simulink model "nldemo_master"  (R2020b)
settings: Solver=FixedStepAuto  StartTime=0.0  StopTime=inf  FixedStep=0.01  RelTol=1e-3
undefined symbols (not defined in the file): autopilot, control, kspTxIn0, P_m_rocket, P_x_target
libraries: ksplib x3
settings Model: DataDictionary=kspdemo.sldd  EnablePacing=on  PacingRate=2  Creator=brianhannan  LastModifiedBy=wizard

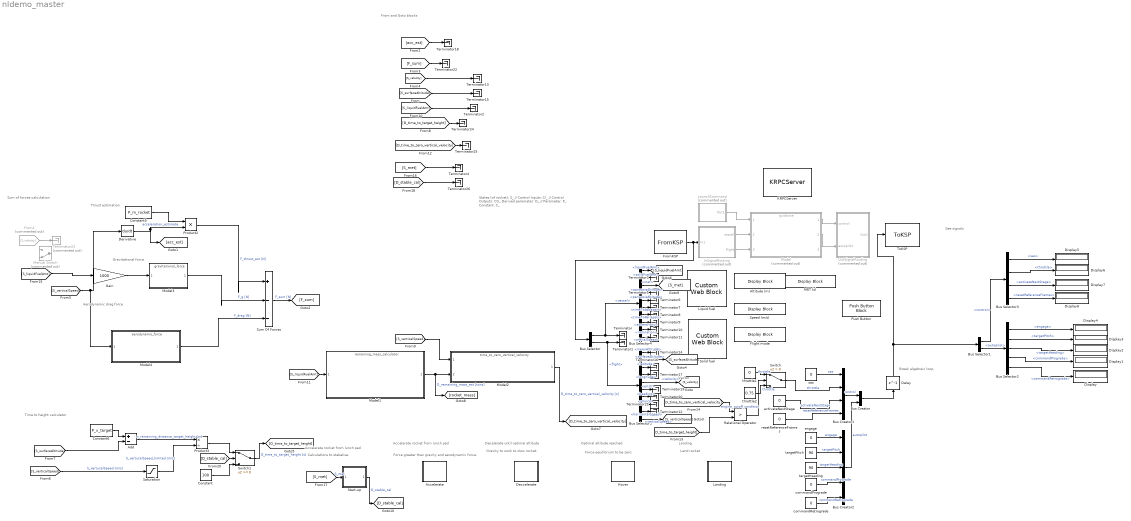
== system nldemo_master ==
  note: Time to height calculator
  note: Vector
  note: From and Goto blocks
  note: Thrust estimation
  note: States (of rocket): 		S_         //
      | Control Inputs: 		CI_       //
      | Control Outputs:		CO_
      | Derived parameter: 	D_     //
      | Parameter:				P_
      | Constant:				C_
  note: Gravitational force
  note: Sum of forces calculation
  note: Gravity to work to slow rocket.
  note: Decelerate until optimal altitude
  note: See signals
  note: Break algebraic loop
  note: Optimal altitude reached
  note: Accelerate rocket from lunch pad
  note: Force greater than gravity and aerodynamic force.
  note: Force equilibrium to be zero:
  note: Land rocket
  note: Landing
  note: Aerodynamic drag force
  note: Accelerate rocket from lunch pad
  note: Calculations to stabalise.
  Accelerate : Stateflow chart  TreatAsAtomicUnit=on
  Add : Sum  Inputs=+-
  Altitude (m) : DisplayBlock  LabelPosition=Bottom  Format=short  Transparency=1
  Bus Creator : BusCreator  Inputs=2  OutDataTypeStr=Bus: kspTxIn  NonVirtualBus=on
  Bus Creator1 : BusCreator  Inputs=4  OutDataTypeStr=Bus: control  NonVirtualBus=on
  Bus Creator2 : BusCreator  Inputs=5  OutDataTypeStr=Bus: autopilot  NonVirtualBus=on
  Bus Selector : BusSelector  OutputSignals=vessel,flight
  Bus Selector1 : BusSelector  OutputSignals=control,autopilot
  Bus Selector2 : BusSelector  OutputSignals=engage,targetPitch,targetHeading,commandPrograde,commandRetrograde
  Bus Selector3 : BusSelector  OutputSignals=sas,throttle,activateNextStage,resetReferenceFrames
  Bus Selector4 : BusSelector  OutputSignals=liquidFuelAmt,solidFuelAmt,met,apoapsisAltitude,periapsisAltitude,timeToApoapsis,timeToPeriapsis,eccentricity,inclination,orbitalSpeed
  Bus Selector5 : BusSelector  OutputSignals=meanAltitude,surfaceAltitude,latitude,longitude,velocity,pitch,heading,gForce,horizontalSpeed,verticalSpeed
  Constant : Constant  Value=100
  Constant5 : Constant  Value=P_m_rocket
  Constant6 : Constant  Value=P_x_target
  "Deccelerate " : Stateflow chart  TreatAsAtomicUnit=on
  Delay : Delay  DelayLength=1
  Derivative : Derivative
  Display{,1..8} (9 alike) : Display
  Flight mode : DisplayBlock  LabelPosition=Bottom  Format=short  Transparency=1
  From1 : From  Commented=on  GotoTag=S_velocity
  FromKSP : ksplib/FromKSP
  Gain : Gain  Gain=1000
  Hover : Stateflow chart  TreatAsAtomicUnit=on
  InSignalRouting : Subsystem  Commented=on
  KRPCServer : ksplib/KRPCServer
  Landing : Stateflow chart  TreatAsAtomicUnit=on
  LaunchCommand : Subsystem  Commented=on  mask(Launch Command){launchCmd=logical(0)}
      mask prompts: launchCmd "Launch:"
      mask help: Send launch command
      mask Display: disp('Launch')
  Liquid fuel : CustomWebBlock  LabelPosition=Hide  ShowInitialText=on  Configuration="{\"components\":[{\"name\":\"CircularScaleComponent\",\"settings\":{\"bounds\":{\"max\":225,\"min\":0,\"tickInterval\":\"auto\"},\"direction\":\"cw\",\"flipLimits\":0,\"innerRadius\":0.75,\"internalTickHeightScaleFactor\":1,\"labelColor\":[255,252,199],\"labelFont\":{\"font\":\"Arial\",\"fontSize\":12},\"labelTransparency\":1,\"minorTickHeightScaleFactor\":0.2,\"needleImage\":{\"size\":[1890,567],\"src\":\"data:image\\/svg+xml;base64,PD94bWwgdmVyc2lvbj0iMS4wIiBlbmNvZGluZz0iVVRGLTgiIHN0YW5kYWxvbmU9Im5vIj8+CjxzdmcKICAgeG1sbnM6ZGM9Imh0dHA6Ly9wdXJsLm9yZy9kYy9lbGVtZW50cy8xLjEvIgogICB4bWxuczpjYz0iaHR0cDovL2NyZWF0aXZlY29tbW9ucy5vcmcvbnMjIgogICB4bWxuczpyZGY9Imh0dHA6Ly93d3cudzMub3JnLzE5OTkvMDIvMjItcmRmLXN5bnRheC1ucyMiCiAgIHhtbG5zOnN2Zz0iaHR0cDovL3d3dy53My5vcmcvMjAwMC9zdmciCiAgIHhtbG5zPSJodHRwOi8vd3d3LnczLm9yZy8yMDAwL3N2ZyIKICAgeG1sbnM6 ...(+4096 chars)\"},\"needleOffset\":[0.1610917094974375,0],\"needleOrientation\":-45,\"needleRotation\":180.59702388394928,\"needleSize\":{\"height\":0.13032601008944536,\"width\":0.416859542883425},\"outerRadius\":0.9,\"position\":[0.06486742424242424,0.05627705627705628,0.8917748917748918,0.8787878787878788],\"scaleAngle\":270,\"scaleAngleOffset\":135,\"scaleColors\":[],\"scaleColorsSize\":0.2,\"scalePosition\":[0,0,1,1],\"showLabels\":1,\"showMinorTicks\":1,\"showSpanLine\":1,\"showTicks\":1,\"tickColor\":[255,255,200],\"tickTransparency\":1,\"valueBarColor\":[0,114,189],\"valueBarPosition\":[0,0,1,1],\"valueBarSize\":0.2,\"valueBarTransparency\":1}},{\"name\":\"BackgroundImageComponent\",\"settings\":{\"image\":{\"size\":[500,500],\"src\":\"data:image\\/svg+xml;base64,PD94bWwgdmVyc2lvbj0iMS4wIiBlbmNvZGluZz0iVVRGLTgiIHN0YW5kYWxvbmU9Im5vIj8+CjxzdmcKICAgeG1sbnM6ZGM9Imh0dHA6Ly9wdXJsLm9yZy9kYy9lbGVtZW50cy8xLjEvIgogICB4bWxuczpjYz0iaHR0cDovL2NyZWF0aXZlY29tbW9ucy5vcmcvbnMjIgogICB4bWxuczpyZGY9Imh0dHA6Ly93d3cudzMub3JnLzE5OTkvMDIvMjItcmRmLXN5bnRheC1ucyMiCiAgIHhtbG5zOnN2Zz0iaHR0cDovL3d3dy53My5vcmcvMjAwMC9zdmciCiAgIHhtbG5zPSJodHRwOi8vd3d3LnczLm9yZy8yMDAwL3N2ZyIKICAgeG1sbnM6 ...(+9964 chars)\"},\"position\":[0,0,1,1],\"scaleMode\":\"0\"}},{\"name\":\"ForegroundImageComponent\",\"settings\":{\"image\":{\"size\":[0,0],\"src\":\"default\",\"srcOrientation\":[]},\"isForeground\":1,\"position\":[0,0,1,1],\"scaleMode\":\"0\"}}],\"settings\":{\"BindingType\":\"signal\",\"aspectRatio\":1.0318471337579618,\"direction\":\"cw\",\"fixedAspectRatio\":\"on\",\"flipLimits\":0,\"orientation\":\"horizontal\"},\"type\":\"CircularGauge\"}"
  MET (s) : DisplayBlock  LabelPosition=Bottom  Format=short  Transparency=1
  Manual Switch : ManualSwitch  Commented=on  CurrentSetting=0
  Model : ModelReference  Commented=on  ModelNameDialog=guidance  SimulationMode=Normal  ModelReferenceVersion=1.177
  Model1 : ModelReference  ModelNameDialog=remaining_mass_calculator.slx  SimulationMode=Normal  ModelReferenceVersion=1.2
  Model2 : ModelReference  ModelNameDialog=time_to_zero_vertical_velocity.slx  SimulationMode=Normal  ModelReferenceVersion=1.4
  Model3 : ModelReference  ModelNameDialog=gravitational_force.slx  SimulationMode=Normal  ModelReferenceVersion=1.5
  Model4 : ModelReference  ModelNameDialog=aerodynamic_force.slx  SimulationMode=Normal  ModelReferenceVersion=1.5
  OutSignalRouting : Subsystem  Commented=on
  Product2 : Product
  Product3 : Product  Inputs=*/
  Push Button : PushButtonBlock  ButtonText=Launch
  Relational Operator : RelationalOperator  Operator=>  OutDataTypeStr=boolean  RndMeth=Simplest
  Saturation : Saturate  UpperLimit=10000  LowerLimit=0.0001
  Solid fuel : CustomWebBlock  LabelPosition=Hide  ShowInitialText=on  Configuration="{\"components\":[{\"name\":\"CircularScaleComponent\",\"settings\":{\"bounds\":{\"max\":750,\"min\":0,\"tickInterval\":\"auto\"},\"direction\":\"cw\",\"flipLimits\":0,\"innerRadius\":0.75,\"internalTickHeightScaleFactor\":1,\"labelColor\":[255,252,199],\"labelFont\":{\"font\":\"Arial\",\"fontSize\":12},\"labelTransparency\":1,\"minorTickHeightScaleFactor\":0.2,\"needleImage\":{\"size\":[1890,567],\"src\":\"data:image\\/svg+xml;base64,PD94bWwgdmVyc2lvbj0iMS4wIiBlbmNvZGluZz0iVVRGLTgiIHN0YW5kYWxvbmU9Im5vIj8+CjxzdmcKICAgeG1sbnM6ZGM9Imh0dHA6Ly9wdXJsLm9yZy9kYy9lbGVtZW50cy8xLjEvIgogICB4bWxuczpjYz0iaHR0cDovL2NyZWF0aXZlY29tbW9ucy5vcmcvbnMjIgogICB4bWxuczpyZGY9Imh0dHA6Ly93d3cudzMub3JnLzE5OTkvMDIvMjItcmRmLXN5bnRheC1ucyMiCiAgIHhtbG5zOnN2Zz0iaHR0cDovL3d3dy53My5vcmcvMjAwMC9zdmciCiAgIHhtbG5zPSJodHRwOi8vd3d3LnczLm9yZy8yMDAwL3N2ZyIKICAgeG1sbnM6 ...(+4096 chars)\"},\"needleOffset\":[0.1610917094974375,0],\"needleOrientation\":-45,\"needleRotation\":180.59702388394928,\"needleSize\":{\"height\":0.13032601008944536,\"width\":0.416859542883425},\"outerRadius\":0.9,\"position\":[0.06486742424242424,0.05627705627705628,0.8917748917748918,0.8787878787878788],\"scaleAngle\":270,\"scaleAngleOffset\":135,\"scaleColors\":[],\"scaleColorsSize\":0.2,\"scalePosition\":[0,0,1,1],\"showLabels\":1,\"showMinorTicks\":1,\"showSpanLine\":1,\"showTicks\":1,\"tickColor\":[255,255,200],\"tickTransparency\":1,\"valueBarColor\":[0,114,189],\"valueBarPosition\":[0,0,1,1],\"valueBarSize\":0.2,\"valueBarTransparency\":1}},{\"name\":\"BackgroundImageComponent\",\"settings\":{\"image\":{\"size\":[500,500],\"src\":\"data:image\\/svg+xml;base64,PD94bWwgdmVyc2lvbj0iMS4wIiBlbmNvZGluZz0iVVRGLTgiIHN0YW5kYWxvbmU9Im5vIj8+CjxzdmcKICAgeG1sbnM6ZGM9Imh0dHA6Ly9wdXJsLm9yZy9kYy9lbGVtZW50cy8xLjEvIgogICB4bWxuczpjYz0iaHR0cDovL2NyZWF0aXZlY29tbW9ucy5vcmcvbnMjIgogICB4bWxuczpyZGY9Imh0dHA6Ly93d3cudzMub3JnLzE5OTkvMDIvMjItcmRmLXN5bnRheC1ucyMiCiAgIHhtbG5zOnN2Zz0iaHR0cDovL3d3dy53My5vcmcvMjAwMC9zdmciCiAgIHhtbG5zPSJodHRwOi8vd3d3LnczLm9yZy8yMDAwL3N2ZyIKICAgeG1sbnM6 ...(+9964 chars)\"},\"position\":[0,0,1,1],\"scaleMode\":\"0\"}},{\"name\":\"ForegroundImageComponent\",\"settings\":{\"image\":{\"size\":[0,0],\"src\":\"default\",\"srcOrientation\":[]},\"isForeground\":1,\"position\":[0,0,1,1],\"scaleMode\":\"0\"}}],\"settings\":{\"BindingType\":\"signal\",\"aspectRatio\":1.0318471337579618,\"direction\":\"cw\",\"fixedAspectRatio\":\"on\",\"flipLimits\":0,\"orientation\":\"horizontal\"},\"type\":\"CircularGauge\"}"
  Speed (m/s) : DisplayBlock  LabelPosition=Bottom  Format=short  Transparency=1
  Start-up : Stateflow chart  TreatAsAtomicUnit=on
  Sum Of Forces : Sum  Inputs=|+--
  Switch : Switch  Criteria=u2 > Threshold
  Switch1 : Switch
  Terminator{,1..22,24..26} (26 alike) : Terminator
  Terminator23 : Terminator  Commented=on
  ToKSP : ksplib/ToKSP
  activateNextStage : Constant  Value=0  OutDataTypeStr=boolean
  commandPrograde : Constant  Value=0  OutDataTypeStr=boolean
  commandRetrograde : Constant  Value=0  OutDataTypeStr=boolean
  engage : Constant  Value=0  OutDataTypeStr=boolean
  resetReferenceFrames : Constant  Value=0  OutDataTypeStr=boolean
  sas : Constant  Value=0  OutDataTypeStr=boolean
  targetHeading : Constant  Value=90
  targetPitch : Constant  Value=90
  throttle1 : Constant  Value=0
  throttle2 : Constant  Value=0.75
  wires:
  LaunchCommand/1(Out1) -> Model/1
  Model/1 -> OutSignalRouting/1(control)
  Model/2 -> OutSignalRouting/2(autopilot)
  Bus Creator/1 -> Delay/1
  FromKSP/1 -> InSignalRouting/1(In1), Bus Selector/1
  InSignalRouting/1(vessel) -> Model/2
  InSignalRouting/2(flight) -> Model/3
  Bus Selector/2 -> Bus Selector5/1, Terminator1/1  "<flight>"
  Bus Selector/1 -> Bus Selector4/1, Terminator/1  "<vessel>"
  Switch/1 -> Bus Creator1/2  "throttle"
  engage/1 -> Bus Creator2/1  "engage"
  targetPitch/1 -> Bus Creator2/2  "targetPitch"
  targetHeading/1 -> Bus Creator2/3  "targetHeading"
  Bus Creator2/1 -> Bus Creator/2  "autopilot"
  Bus Creator1/1 -> Bus Creator/1  "control"
  sas/1 -> Bus Creator1/1  "sas"
  activateNextStage/1 -> Bus Creator1/3  "activateNextStage"
  commandRetrograde/1 -> Bus Creator2/5  "commandRetrograde"
  commandPrograde/1 -> Bus Creator2/4  "commandPrograde"
  Bus Selector2/2 -> Display3/1  "<targetPitch>"
  Bus Selector2/3 -> Display2/1  "<targetHeading>"
  Bus Selector1/2 -> Bus Selector2/1  "<autopilot>"
  Bus Selector2/5 -> Display/1  "<commandRetrograde>"
  Bus Selector2/1 -> Display4/1  "<engage>"
  Delay/1 -> Bus Selector1/1, ToKSP/1
  Bus Selector2/4 -> Display1/1  "<commandPrograde>"
  Bus Selector3/4 -> Display8/1  "<resetReferenceFrames>"
  Bus Selector3/3 -> Display7/1  "<activateNextStage>"
  Bus Selector1/1 -> Bus Selector3/1  "<control>"
  Bus Selector3/2 -> Display6/1  "<throttle>"
  Bus Selector3/1 -> Display5/1  "<sas>"
  resetReferenceFrames/1 -> Bus Creator1/4  "resetReferenceFrames"
  Bus Selector4/1 -> [S_liquidFuelAmt]  "<liquidFuelAmt>"
  Bus Selector4/2 -> Terminator3/1  "<solidFuelAmt>"
  Bus Selector4/3 -> [S_met]  "<met>"
  Bus Selector4/4 -> Terminator5/1  "<apoapsisAltitude>"
  Bus Selector4/5 -> Terminator6/1  "<periapsisAltitude>"
  Bus Selector4/6 -> Terminator7/1  "<timeToApoapsis>"
  Bus Selector4/7 -> Terminator8/1  "<timeToPeriapsis>"
  Bus Selector4/8 -> Terminator9/1  "<eccentricity>"
  Bus Selector4/9 -> Terminator10/1  "<inclination>"
  Bus Selector4/10 -> Terminator11/1  "<orbitalSpeed>"
  Bus Selector5/1 -> Terminator14/1  "<meanAltitude>"
  Bus Selector5/2 -> [S_surfaceAltitude]  "<surfaceAltitude>"
  Bus Selector5/3 -> Terminator16/1  "<latitude>"
  Bus Selector5/4 -> Terminator17/1  "<longitude>"
  Bus Selector5/5 -> [S_velocity]  "<velocity>"
  Bus Selector5/6 -> Terminator19/1  "<pitch>"
  Bus Selector5/7 -> Terminator20/1  "<heading>"
  Bus Selector5/8 -> Terminator21/1  "<gForce>"
  Bus Selector5/9 -> Terminator12/1  "<horizontalSpeed>"
  Bus Selector5/10 -> [S_verticalSpeed]  "<verticalSpeed>"
  [S_verticalSpeed] -> Model4/1, Derivative/1
  From1/1 -> Terminator23/1
  Derivative/1 -> Product2/2, [acc_est]  "acceleration_estimate"
  Constant5/1 -> Product2/1
  Product2/1 -> Sum Of Forces/1  "F_thrust_est [N]"
  [acc_est] -> Terminator18/1
  Sum Of Forces/1 -> [F_sum]  "F_sum [N]"
  [F_sum] -> Terminator22/1
  [S_velocity] -> Terminator13/1
  Constant6/1 -> Add/1
  [S_surfaceAltitude] -> Terminator15/1
  [S_surfaceAltitude] -> Add/2
  Add/1 -> Product3/1  "x_remaining_distance_target_height [m]"
  [S_verticalSpeed] -> Saturation/1  "S_vertucalSpeed [m/s]"
  Saturation/1 -> Product3/2  "S_vertucalSpeed_limited [m/s]"
  Switch1/1 -> [D_time_to_target_height]  "D_time_to_target_height [s]"
  [D_time_to_target_height] -> Terminator24/1
  Model3/1 -> Sum Of Forces/2  "F_g [N]"
  [S_verticalSpeed] -> Model2/1
  Model1/1 -> [rocket_mass], Model2/2  "D_remaining_mass_est [tons]"
  [S_liquidFuelAmt] -> Terminator2/1
  [S_liquidFuelAmt] -> Model1/1
  Model2/1 -> [D_time_to_zero_vertical_velocity]  "D_time_to_zero_vertical_velocity [s]"
  [D_time_to_zero_vertical_velocity] -> Terminator25/1
  Model4/1 -> Sum Of Forces/3  "F_drag [N]"
  [D_time_to_target_height] -> Relational Operator/2
  [D_time_to_zero_vertical_velocity] -> Relational Operator/1
  throttle2/1 -> Switch/3  "throttle"
  throttle1/1 -> Switch/1  "throttle"
  Relational Operator/1 -> Switch/2  "engine_cutoff_condition"
  [S_liquidFuelAmt] -> Gain/1
  Gain/1 -> Model3/1
  [S_met] -> Terminator4/1
  [S_met] -> Start-up/1(S_met)  "S_met"
  Start-up/1(D_stable_cal) -> [D_stable_cal]  "D_stable_cal"
  [D_stable_cal] -> Terminator26/1
  [D_stable_cal] -> Switch1/2
  Product3/1 -> Switch1/1
  Constant/1 -> Switch1/3

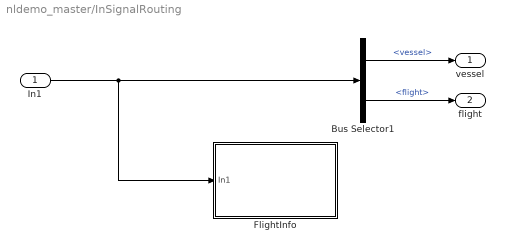
== system nldemo_master/InSignalRouting ==
  In1 : Inport
  Bus Selector1 : BusSelector  OutputSignals=vessel,flight
  FlightInfo : Subsystem
  vessel : Outport
  flight : Outport  Port=2
  wires:
  Bus Selector1/1 -> vessel/1  "<vessel>"
  Bus Selector1/2 -> flight/1  "<flight>"
  In1/1 -> FlightInfo/1(In1), Bus Selector1/1

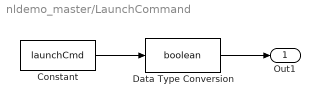
== system nldemo_master/LaunchCommand ==
  Constant : Constant  Value=launchCmd
  Data Type Conversion : DataTypeConversion  OutDataTypeStr=boolean
  Out1 : Outport
  wires:
  Constant/1 -> Data Type Conversion/1
  Data Type Conversion/1 -> Out1/1

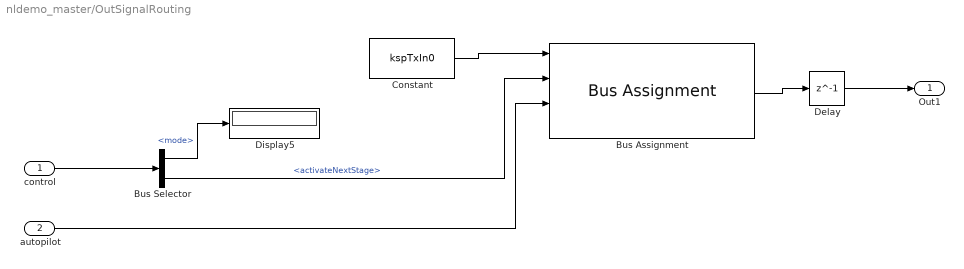
== system nldemo_master/OutSignalRouting ==
  control : Inport  OutDataTypeStr=Bus: mcout
  autopilot : Inport  Port=2  OutDataTypeStr=Bus: autopilot
  Bus Assignment : BusAssignment  AssignedSignals=control.activateNextStage,autopilot,control.throttle
  Bus Selector : BusSelector  OutputSignals=mode,activateNextStage
  Constant : Constant  Value=kspTxIn0  OutDataTypeStr=Bus: kspTxIn
  Delay : Delay  DelayLength=1
  Display5 : Display
  Out1 : Outport
  wires:
  Bus Assignment/1 -> Delay/1
  autopilot/1 -> Bus Assignment/3
  control/1 -> Bus Selector/1
  Bus Selector/2 -> Bus Assignment/2  "<activateNextStage>"
  Constant/1 -> Bus Assignment/1
  Bus Selector/1 -> Display5/1  "<mode>"
  Delay/1 -> Out1/1

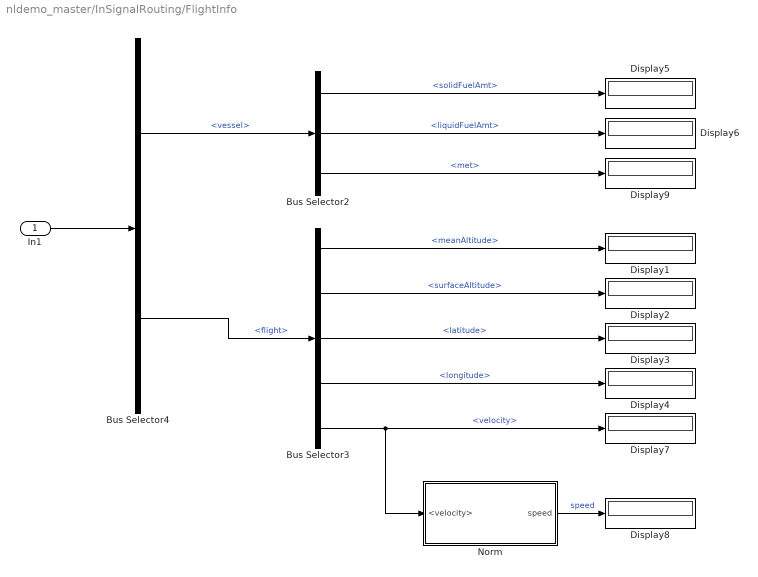
== system nldemo_master/InSignalRouting/FlightInfo ==
  In1 : Inport
  Bus Selector2 : BusSelector  OutputSignals=solidFuelAmt,liquidFuelAmt,met
  Bus Selector3 : BusSelector  OutputSignals=meanAltitude,surfaceAltitude,latitude,longitude,velocity
  Bus Selector4 : BusSelector  OutputSignals=vessel,flight
  Display{1..9} (9 alike) : Display
  Norm : Subsystem
  wires:
  Bus Selector2/2 -> Display6/1  "<liquidFuelAmt>"
  In1/1 -> Bus Selector4/1
  Bus Selector3/2 -> Display2/1  "<surfaceAltitude>"
  Bus Selector4/2 -> Bus Selector3/1  "<flight>"
  Bus Selector4/1 -> Bus Selector2/1  "<vessel>"
  Bus Selector3/4 -> Display4/1  "<longitude>"
  Bus Selector3/3 -> Display3/1  "<latitude>"
  Bus Selector3/1 -> Display1/1  "<meanAltitude>"
  Bus Selector2/1 -> Display5/1  "<solidFuelAmt>"
  Bus Selector3/5 -> Norm/1(<velocity>), Display7/1  "<velocity>"
  Norm/1(speed) -> Display8/1  "speed"
  Bus Selector2/3 -> Display9/1  "<met>"

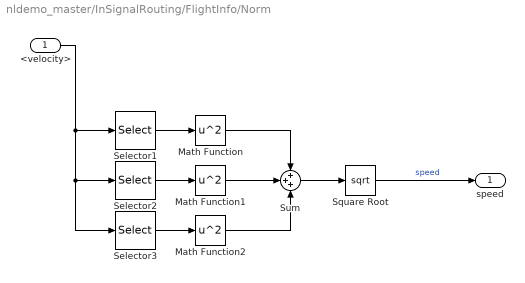
== system nldemo_master/InSignalRouting/FlightInfo/Norm ==
  <velocity> : Inport
  Math Function : Math  Operator=square  SaturateOnIntegerOverflow=on
  Math Function1 : Math  Operator=square  SaturateOnIntegerOverflow=on
  Math Function2 : Math  Operator=square  SaturateOnIntegerOverflow=on
  Selector1 : Selector  InputPortWidth=3  IndexOptions=Index vector (dialog)  Indices=1  OutputSizes=1
  Selector2 : Selector  InputPortWidth=3  IndexOptions=Index vector (dialog)  Indices=2  OutputSizes=1
  Selector3 : Selector  InputPortWidth=3  IndexOptions=Index vector (dialog)  Indices=3  OutputSizes=1
  Square Root : Sqrt  SaturateOnIntegerOverflow=on
  Sum : Sum  Inputs=+++
  speed : Outport
  wires:
  Square Root/1 -> speed/1  "speed"
  Selector1/1 -> Math Function/1
  Sum/1 -> Square Root/1
  Math Function2/1 -> Sum/3
  Math Function/1 -> Sum/1
  Math Function1/1 -> Sum/2
  Selector2/1 -> Math Function1/1
  Selector3/1 -> Math Function2/1
  <velocity>/1 -> Selector3/1, Selector2/1, Selector1/1

== stateflow chart nldemo_master/Deccelerate  ==

== stateflow chart nldemo_master/Start-up ==
  state StartCalculations
    entry: D_stable_cal = 0;
  state StabilCalculations
    entry: D_stable_cal = 1;
  (default) -> StartCalculations
  StartCalculations -> StabilCalculations : [S_met > 2]
  data: S_met input; D_stable_cal output

== stateflow chart nldemo_master/Accelerate ==

== stateflow chart nldemo_master/Landing ==

== stateflow chart nldemo_master/Hover ==
